simulink model "asbQuadcopter"  (R2025b)
settings: Solver=ode3  StartTime=0  StopTime=20  FixedStep=Ts  RelTol=1e-3  EnableMultiTasking=on
undefined symbols (not defined in the file): Command, ft, init, m, Rec, s, SDTV, Sim3dSensor, takeOffDuration, Ts, Vehicle
libraries: simulink x18, sim3dlib x6, aerolibconvert2 x5, aerolibsim3d x4, aerolibanimutils x2, SignalEditorBlockLib x2, environmentLibrary x2, visionconversions x2, visiongeotforms x2, visionsinks x2, sensorsLibrary x2, aerolibfltsims x2
(part 1 of 2)
settings Model: Creator=The MathWorks, Inc.  LastModifiedBy=poiuy
settings SolverCC: AlgebraicLoopSolver=TrustRegion  AutoInsertRateTranBlk=on  MaxZcPerStep=1.0
settings DataIOCC: LimitDataPoints=on  SaveFormat=Array  SaveOutput=off  DSMLogging=off  SaveTime=off  ReturnWorkspaceOutputs=off
settings OptimizationCC: BlockReduction=off  BufferReuse=off  ReuseModelBlockBuffer=off  LifeSpan=inf
settings DebuggingCC: AlgebraicLoopMsg=none  ParameterPrecisionLossMsg=none  AllowSymbolicDim=off  PregeneratedLibrarySubsystemCodeDiagnostic=none  SFUnexpectedBacktrackingDiag=warning  SFNoUnconditionalDefaultTransitionDiag=warning  SFExecutionAtInitializationDiag=none  ArithmeticOperatorsInVariantConditions=warning
settings HardwareCC: ProdBitPerPointer=32.0  ProdBitPerSizeT=32.0  ProdBitPerPtrDiffT=32.0  ProdLargestAtomicFloat=None  ProdIntDivRoundTo=Undefined  ProdEndianess=Unspecified  ProdWordSize=32.0  ProdHWDeviceType=32-bit Generic
settings ModelReferenceCC: EnableRefExpFcnMdlSchedulingChecks=on  PropagateSignalLabelsOutOfModel=off
settings SFSimCC: SimUseLocalCustomCode=off  CustomCodeUndefinedFunction=UseInterfaceOnly
settings RTWCC: RTWUseLocalCustomCode=off  GPUComputeCapability=3.5  DLArmComputeVersion=19.05
settings CodeAppCC: StateflowObjectComments=on
settings GRTTargetCC: TargetLangStandard=C89/C90 (ANSI)
settings ConfigComp: CovMetricSettings=dw  CovSaveCumulativeToWorkspaceVar=on  CovSaveSingleToWorkspaceVar=on  CovExternalEMLEnable=off  CovSFcnEnable=off

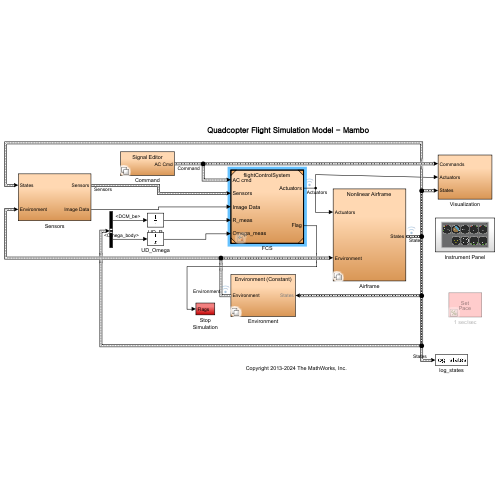
[thumbnail: Simulink's stored preview of the top-level diagram]
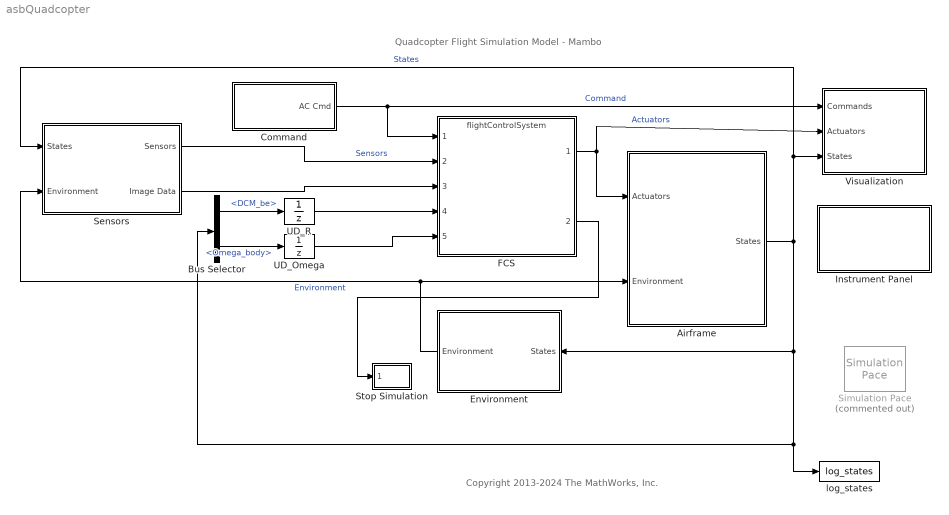
== system asbQuadcopter ==
  note: Quadcopter Flight Simulation Model - Mambo
  note: Copyright 2013-2024 The MathWorks, Inc.
  Airframe : Subsystem  Variant=on
  Bus Selector : BusSelector  OutputSignals=DCM_be,Omega_body
  Command : Subsystem  Variant=on
  Environment : Subsystem  Variant=on
  FCS : ModelReference  ModelNameDialog=flightControlSystem.slx  SimulationMode=Normal  ModelReferenceVersion=13.7
  Instrument Panel : Subsystem
  Sensors : Subsystem
  Simulation Pace : aerolibanimutils/Simulation Pace  Commented=on  SimulationPace=1  SleepMode=MATLAB Thread  OutputPaceError=off  SampleTime=Ts
      settings: AttributesFormatString=%<SimulationPace> sec/sec
  Stop Simulation : Subsystem
  UD_Omega : UnitDelay  SampleTime=0.005  HasFrameUpgradeWarning=on
  UD_R : UnitDelay  SampleTime=0.005  HasFrameUpgradeWarning=on
  Visualization : Subsystem
  log_states : ToWorkspace  VariableName=log_states  SaveFormat=Timeseries  SampleTime=-1
  wires:
  Command/1(AC Cmd) -> Visualization/1(Commands), FCS/1  "Command"
  Sensors/1(Sensors) -> FCS/2  "Sensors"
  FCS/1 -> Airframe/1(Actuators), Visualization/2(Actuators)  "Actuators"
  Environment/1(Environment) -> Sensors/2(Environment), Airframe/2(Environment)  "Environment"
  Sensors/2(Image Data) -> FCS/3
  Bus Selector/2 -> UD_Omega/1  "<Omega_body>"
  UD_Omega/1 -> FCS/5
  UD_R/1 -> FCS/4
  Bus Selector/1 -> UD_R/1  "<DCM_be>"
  FCS/2 -> Stop Simulation/1(Flags)
  Airframe/1(States) -> Environment/1(States), log_states/1, Bus Selector/1, Visualization/3(States), Sensors/1(States)  "States"

== system asbQuadcopter/Airframe ==
  note: VSS_VEHICLE = 0 will select linear airframe
      | VSS_VEHICLE = 1 will select nonlnear airframe
  Actuators : Inport
  Environment : Inport  Port=2  OutDataTypeStr=Bus: EnvironmentBus
  Linear Airframe : ModelReference  ModelNameDialog=linearAirframe.slx  SimulationMode=Normal  VariantControl=VSS_VEHICLE==DynamicsMode.Linear  ModelReferenceVersion=13.0
  Nonlinear Airframe : ModelReference  ModelNameDialog=nonlinearAirframe.slx  SimulationMode=Normal  VariantControl=VSS_VEHICLE==DynamicsMode.Nonlinear  ModelReferenceVersion=13.60
  States : Outport  OutDataTypeStr=Bus: StatesBus  VectorParamsAs1DForOutWhenUnconnected=off

== system asbQuadcopter/Command ==
  note: VSS_COMMAND = 0 will select Signal Editor
      | VSS_COMMAND = 1 will select Joystick + Signal Editor
      | VSS_COMMAND = 2 will select pre-saved data from .mat file
      | VSS_COMMAND = 3 will select pre-saved data from a spreadsheet
  Data : Subsystem  VariantControl=VSS_COMMAND==CommandMode.Presaved_data
  Joystick : Subsystem  VariantControl=VSS_COMMAND==CommandMode.Joystick
  Signal Editor : Subsystem  VariantControl=VSS_COMMAND==CommandMode.Signal_Editor
  Spreadsheet Data : Subsystem  VariantControl=VSS_COMMAND==CommandMode.Presaved_data_in_a_Spreadsheet
  AC Cmd : Outport  OutDataTypeStr=Bus: CommandBus  VectorParamsAs1DForOutWhenUnconnected=off

== system asbQuadcopter/Environment ==
  note: VSS_ENVIRONMENT = 0 will select constant environment variables
      | VSS_ENVIRONMENT = 1 will select environment variables depending on position
  States : Inport  OutDataTypeStr=Bus: StatesBus
  Environment (Constant) : environmentLibrary/Environment (Constant)  SystemSampleTime=-1  VariantControl=VSS_ENVIRONMENT==EnvironmentMode.Constant  VariantActivationTime=update diagram  EmptyChoice=off  PassThrough=off  PassThroughVariantControl=(default)  EmptyChoiceVariantControl=(default)  AllowFlexibleInterface=on  Latency=0  AutoFrameSizeCalculation=off
  Environment (Variable) : environmentLibrary/Environment (Variable)  SystemSampleTime=-1  VariantControl=VSS_ENVIRONMENT==EnvironmentMode.Variable  VariantActivationTime=update diagram  EmptyChoice=off  PassThrough=off  PassThroughVariantControl=(default)  EmptyChoiceVariantControl=(default)  AllowFlexibleInterface=on  Latency=0  AutoFrameSizeCalculation=off
  Environment : Outport  OutDataTypeStr=Bus: EnvironmentBus  VectorParamsAs1DForOutWhenUnconnected=off

== system asbQuadcopter/Instrument Panel ==
  Airspeed Indicator : AirspeedIndicatorBlock  LabelPosition=Hide  ScaleMin=0  ScaleMax=18
  Altimeter : AltimeterBlock  LabelPosition=Hide
  Artificial Horizon : ArtificialHorizonBlock  LabelPosition=Hide
  Climb Rate Indicator : ClimbIndicatorBlock  LabelPosition=Hide  ScaleMax=1000
  Heading Indicator : HeadingIndicatorBlock  LabelPosition=Hide
  Thruster {1..4} (4 alike) : RPMIndicatorBlock  LabelPosition=Hide

== system asbQuadcopter/Sensors ==
  States : Inport
  Environment : Inport  Port=2
  Camera Model : Subsystem  Variant=on
  Rate Transition3 : RateTransition  InitialCondition=zeros(4,9600)  OutPortSampleTime=VTs
  Sensor Model : Subsystem  Variant=on
  Sensors : Outport
  Image Data : Outport  Port=2
  wires:
  States/1 -> Sensor Model/1(States)
  Environment/1 -> Sensor Model/2(Environment)
  Sensor Model/1(Sensors) -> Sensors/1  "Sensors"
  Camera Model/1(image_data) -> Rate Transition3/1
  Rate Transition3/1 -> Image Data/1

== system asbQuadcopter/Stop Simulation ==
  Flags : Inport  OutDataTypeStr=uint8
  Compare To Zero : simulink/Logic and Bit Operations/Compare To Zero  relop=>  OutDataTypeStr=boolean
  Flag has been triggered : Assertion  Enabled=off
  Logical Operator : Logic  Operator=NOT  AllPortsSameDT=off  OutDataTypeStr=boolean
  wires:
  Flags/1 -> Compare To Zero/1
  Logical Operator/1 -> Flag has been triggered/1
  Compare To Zero/1 -> Logical Operator/1

== system asbQuadcopter/Visualization ==
  Commands : Inport
  Actuators : Inport  Port=2
  States : Inport  Port=3
  "Actuators " : InportShadow  Port=2
  Extract Flight Instruments : Subsystem
  "States " : InportShadow  Port=3
  Visualization : Subsystem  Variant=on
  wires:
  Actuators/1 -> Extract Flight Instruments/1(Actuators)
  States/1 -> Extract Flight Instruments/2(States)
  Commands/1 -> Visualization/2(Commands)
  "Actuators "/1 -> Visualization/3(Actuators)
  "States "/1 -> Visualization/1(States)

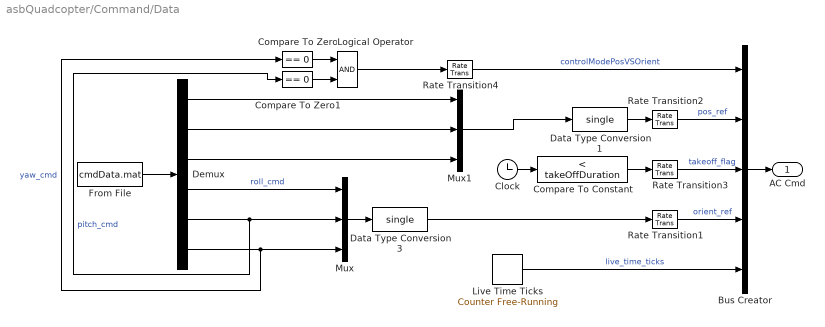
== system asbQuadcopter/Command/Data ==
  Bus Creator : BusCreator  Inputs=5  OutDataTypeStr=Bus: CommandBus  NonVirtualBus=on
  Clock : Clock
  Compare To Constant : simulink/Logic and Bit Operations/Compare To Constant  relop=<  const=takeOffDuration  OutDataTypeStr=boolean
  Compare To Zero : simulink/Logic and Bit Operations/Compare To Zero  relop===  OutDataTypeStr=boolean
  Compare To Zero1 : simulink/Logic and Bit Operations/Compare To Zero  relop===  OutDataTypeStr=boolean
  Data Type Conversion1 : DataTypeConversion  OutDataTypeStr=single  SaturateOnIntegerOverflow=off  RndMeth=Floor
  Data Type Conversion3 : DataTypeConversion  OutDataTypeStr=single  SaturateOnIntegerOverflow=off  RndMeth=Floor
  Demux : Demux  Outputs=6
  From File : FromFile  FileName=cmdData.mat  SampleTime=Ts
  Live Time Ticks : simulink/Sources/Counter Free-Running  NumBits=32  tsamp=Ts
  Logical Operator : Logic  AllPortsSameDT=off  OutDataTypeStr=boolean
  Mux : Mux  Inputs=3
  Mux1 : Mux  Inputs=3
  Rate Transition{1..4} (4 alike) : RateTransition  OutPortSampleTime=Ts
  AC Cmd : Outport  OutDataTypeStr=Bus: CommandBus  VectorParamsAs1DForOutWhenUnconnected=off
  wires:
  Demux/4 -> Mux/1  "roll_cmd"
  Demux/5 -> Mux/2, Compare To Zero1/1  "pitch_cmd"
  Demux/6 -> Compare To Zero/1, Mux/3  "yaw_cmd"
  From File/1 -> Demux/1
  Logical Operator/1 -> Rate Transition4/1
  Rate Transition1/1 -> Bus Creator/4  "orient_ref"
  Rate Transition2/1 -> Bus Creator/2  "pos_ref"
  Demux/3 -> Mux1/3
  Mux/1 -> Data Type Conversion3/1
  Data Type Conversion1/1 -> Rate Transition2/1
  Demux/1 -> Mux1/1
  Compare To Zero1/1 -> Logical Operator/2
  Compare To Zero/1 -> Logical Operator/1
  Mux1/1 -> Data Type Conversion1/1
  Clock/1 -> Compare To Constant/1
  Rate Transition4/1 -> Bus Creator/1  "controlModePosVSOrient"
  Data Type Conversion3/1 -> Rate Transition1/1
  Demux/2 -> Mux1/2
  Compare To Constant/1 -> Rate Transition3/1
  Rate Transition3/1 -> Bus Creator/3  "takeoff_flag"
  Live Time Ticks/1 -> Bus Creator/5  "live_time_ticks"
  Bus Creator/1 -> AC Cmd/1

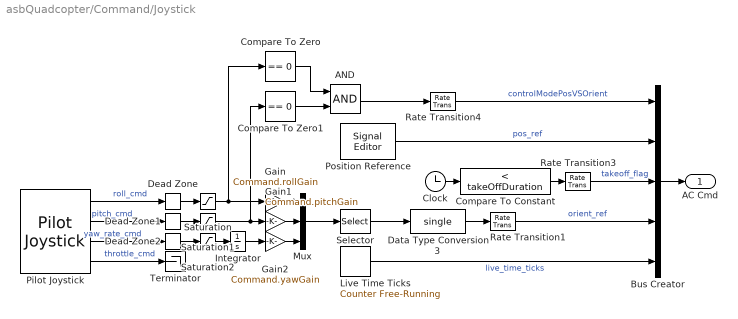
== system asbQuadcopter/Command/Joystick ==
  AND : Logic  AllPortsSameDT=off  OutDataTypeStr=boolean
  Bus Creator : BusCreator  Inputs=5  OutDataTypeStr=Bus: CommandBus  NonVirtualBus=on
  Clock : Clock
  Compare To Constant : simulink/Logic and Bit Operations/Compare To Constant  relop=<  const=takeOffDuration  OutDataTypeStr=boolean
  Compare To Zero : simulink/Logic and Bit Operations/Compare To Zero  relop===  OutDataTypeStr=boolean
  Compare To Zero1 : simulink/Logic and Bit Operations/Compare To Zero  relop===  OutDataTypeStr=boolean
  Data Type Conversion3 : DataTypeConversion  OutDataTypeStr=single  SaturateOnIntegerOverflow=off  RndMeth=Floor
  Dead Zone : DeadZone  LowerValue=Command.rollDeadZoneStart  UpperValue=Command.rollDeadZoneEnd
  Dead Zone1 : DeadZone  LowerValue=Command.pitchDeadZoneStart  UpperValue=Command.pitchDeadZoneEnd
  Dead Zone2 : DeadZone  LowerValue=Command.yawDeadZoneStart  UpperValue=Command.yawDeadZoneEnd
  Gain : Gain  Gain=Command.rollGain
  Gain1 : Gain  Gain=Command.pitchGain
  Gain2 : Gain  Gain=Command.yawGain
  Integrator : Integrator
  Live Time Ticks : simulink/Sources/Counter Free-Running  NumBits=32  tsamp=Ts
  Mux : Mux  Inputs=3
  Pilot Joystick : aerolibanimutils/Pilot Joystick  JoystickID=Joystick1  OutputConfiguration=FourAxis  SampleTime=Ts
  Position Reference : SignalEditorBlockLib/Signal Editor  FileName=positionRef.mat  ActiveScenario=Group1  ActiveSignal=XYZ  IsBus=off  OutputBusObjectStr=Bus: BusObject  SampleTime=Ts  Interpolate=off  ZeroCross=off  OutputAfterFinalValue=Setting to zero  Unit=inherit  PreserveSignalName=on  ApplySigPropsToAllScenarios=on  ApplySigPropsToAllSignals=off  SignalPropertySource=Dialog parameters
  Rate Transition1 : RateTransition  OutPortSampleTime=Ts
  Rate Transition3 : RateTransition  OutPortSampleTime=Ts
  Rate Transition4 : RateTransition  OutPortSampleTime=Ts
  Saturation : Saturate  UpperLimit=Command.rollSatUpper  LowerLimit=Command.rollSatLower
  Saturation1 : Saturate  UpperLimit=Command.pitchSatUpper  LowerLimit=Command.pitchSatLower
  Saturation2 : Saturate  UpperLimit=Command.yawSatUpper  LowerLimit=Command.yawSatLower
  Selector : Selector  InputPortWidth=3  IndexOptions=Index vector (dialog)  Indices=[3 2 1]  OutputSizes=1
  Terminator : Terminator
  AC Cmd : Outport  OutDataTypeStr=Bus: CommandBus  VectorParamsAs1DForOutWhenUnconnected=off
  wires:
  Pilot Joystick/4 -> Terminator/1  "throttle_cmd"
  Pilot Joystick/1 -> Dead Zone/1  "roll_cmd"
  Bus Creator/1 -> AC Cmd/1
  AND/1 -> Rate Transition4/1
  Rate Transition1/1 -> Bus Creator/4  "orient_ref"
  Position Reference/1 -> Bus Creator/2  "pos_ref"
  Mux/1 -> Selector/1
  Compare To Constant/1 -> Rate Transition3/1
  Clock/1 -> Compare To Constant/1
  Rate Transition4/1 -> Bus Creator/1  "controlModePosVSOrient"
  Data Type Conversion3/1 -> Rate Transition1/1
  Pilot Joystick/2 -> Dead Zone1/1  "pitch_cmd"
  Rate Transition3/1 -> Bus Creator/3  "takeoff_flag"
  Live Time Ticks/1 -> Bus Creator/5  "live_time_ticks"
  Selector/1 -> Data Type Conversion3/1
  Dead Zone/1 -> Saturation/1
  Saturation/1 -> Compare To Zero/1, Gain/1
  Gain/1 -> Mux/1
  Dead Zone1/1 -> Saturation1/1
  Saturation1/1 -> Compare To Zero1/1, Gain1/1
  Gain1/1 -> Mux/2
  Dead Zone2/1 -> Saturation2/1
  Saturation2/1 -> Integrator/1
  Gain2/1 -> Mux/3
  Pilot Joystick/3 -> Dead Zone2/1  "yaw_rate_cmd"
  Integrator/1 -> Gain2/1
  Compare To Zero/1 -> AND/1
  Compare To Zero1/1 -> AND/2

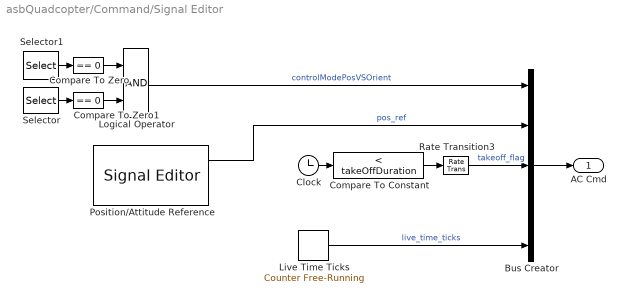
== system asbQuadcopter/Command/Signal Editor ==
  Bus Creator : BusCreator  Inputs=5  OutDataTypeStr=Bus: CommandBus  NonVirtualBus=on
  Clock : Clock
  Compare To Constant : simulink/Logic and Bit Operations/Compare To Constant  relop=<  const=takeOffDuration  OutDataTypeStr=boolean
  Compare To Zero : simulink/Logic and Bit Operations/Compare To Zero  relop===  OutDataTypeStr=boolean
  Compare To Zero1 : simulink/Logic and Bit Operations/Compare To Zero  relop===  OutDataTypeStr=boolean
  Live Time Ticks : simulink/Sources/Counter Free-Running  NumBits=32  tsamp=Ts
  Logical Operator : Logic  AllPortsSameDT=off  OutDataTypeStr=boolean
  Position/Attitude Reference : SignalEditorBlockLib/Signal Editor  FileName=positionAttitudeRef.mat  ActiveScenario=Hover  ActiveSignal=XYZ  IsBus=off  OutputBusObjectStr=Bus: BusObject  SampleTime=Ts  ZeroCross=off  OutputAfterFinalValue=Holding final value  Unit=inherit  PreserveSignalName=on  ApplySigPropsToAllScenarios=on  ApplySigPropsToAllSignals=off  SignalPropertySource=Dialog parameters
  Rate Transition3 : RateTransition  OutPortSampleTime=Ts
  Selector : Selector  InputPortWidth=3  IndexOptions=Index vector (dialog)  Indices=2  OutputSizes=1
  Selector1 : Selector  InputPortWidth=3  IndexOptions=Index vector (dialog)  Indices=3  OutputSizes=1
  AC Cmd : Outport  OutDataTypeStr=Bus: CommandBus  VectorParamsAs1DForOutWhenUnconnected=off
  wires:
  Bus Creator/1 -> AC Cmd/1
  ? -> Bus Creator/4, Selector1/1, Selector/1  "orient_ref"
  Compare To Zero/1 -> Logical Operator/1
  Compare To Zero1/1 -> Logical Operator/2
  Logical Operator/1 -> Bus Creator/1  "controlModePosVSOrient"
  Position/Attitude Reference/1 -> Bus Creator/2  "pos_ref"
  Clock/1 -> Compare To Constant/1
  Compare To Constant/1 -> Rate Transition3/1
  Rate Transition3/1 -> Bus Creator/3  "takeoff_flag"
  Live Time Ticks/1 -> Bus Creator/5  "live_time_ticks"
  Selector/1 -> Compare To Zero1/1
  Selector1/1 -> Compare To Zero/1

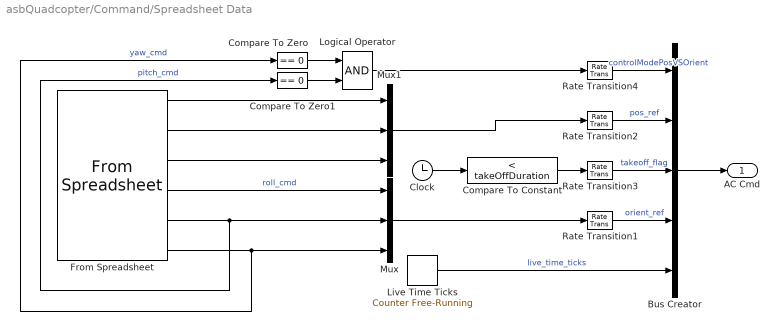
== system asbQuadcopter/Command/Spreadsheet Data ==
  Bus Creator : BusCreator  Inputs=5  OutDataTypeStr=Bus: CommandBus  NonVirtualBus=on
  Clock : Clock
  Compare To Constant : simulink/Logic and Bit Operations/Compare To Constant  relop=<  const=takeOffDuration  OutDataTypeStr=boolean
  Compare To Zero : simulink/Logic and Bit Operations/Compare To Zero  relop===  OutDataTypeStr=boolean
  Compare To Zero1 : simulink/Logic and Bit Operations/Compare To Zero  relop===  OutDataTypeStr=boolean
  From Spreadsheet : FromSpreadsheet  FileName=cmdData.xlsx  SheetName=data  OutDataTypeStr=single  SampleTime=Ts
  Live Time Ticks : simulink/Sources/Counter Free-Running  NumBits=32  tsamp=Ts
  Logical Operator : Logic  AllPortsSameDT=off  OutDataTypeStr=boolean
  Mux : Mux  Inputs=3
  Mux1 : Mux  Inputs=3
  Rate Transition{1..4} (4 alike) : RateTransition  OutPortSampleTime=Ts
  AC Cmd : Outport  OutDataTypeStr=Bus: CommandBus  VectorParamsAs1DForOutWhenUnconnected=off
  wires:
  Bus Creator/1 -> AC Cmd/1
  From Spreadsheet/4 -> Mux/1  "roll_cmd"
  From Spreadsheet/6 -> Mux/3, Compare To Zero/1  "yaw_cmd"
  Logical Operator/1 -> Rate Transition4/1
  Rate Transition1/1 -> Bus Creator/4  "orient_ref"
  Rate Transition2/1 -> Bus Creator/2  "pos_ref"
  From Spreadsheet/3 -> Mux1/3
  Mux1/1 -> Rate Transition2/1
  From Spreadsheet/1 -> Mux1/1
  Compare To Zero1/1 -> Logical Operator/2
  Compare To Zero/1 -> Logical Operator/1
  Compare To Constant/1 -> Rate Transition3/1
  Clock/1 -> Compare To Constant/1
  Rate Transition4/1 -> Bus Creator/1  "controlModePosVSOrient"
  Mux/1 -> Rate Transition1/1
  From Spreadsheet/5 -> Mux/2, Compare To Zero1/1  "pitch_cmd"
  From Spreadsheet/2 -> Mux1/2
  Rate Transition3/1 -> Bus Creator/3  "takeoff_flag"
  Live Time Ticks/1 -> Bus Creator/5  "live_time_ticks"

== system asbQuadcopter/Sensors/Camera Model ==
  note: VSS_VISUALIZATION < 3 will select Camera (Stub)
      | VSS_VISUALIZATION ==3 will select Camera (Airport)
      | VSS_VISUALIZATION ==4 will select Camera (AppleHill)
  Camera (Airport) : Subsystem  VariantControl=VSS_VISUALIZATION==3
  Camera (AppleHill) : Subsystem  VariantControl=VSS_VISUALIZATION==4
  Camera (Stub) : Subsystem  VariantControl=VSS_VISUALIZATION<3
  image_data : Outport

== system asbQuadcopter/Sensors/Sensor Model ==
  note: VSS_SENSORS = 0 will select feedthrough sensors
      | VSS_SENSORS = 1 will select dynamics sensors with noise
  States : Inport
  Environment : Inport  Port=2
  Sensors (Dynamics) : sensorsLibrary/Sensors (Dynamics)  SystemSampleTime=-1  VariantControl=VSS_SENSORS==SensorsMode.Dynamics  VariantActivationTime=update diagram  EmptyChoice=off  PassThrough=off  PassThroughVariantControl=(default)  EmptyChoiceVariantControl=(default)  AllowFlexibleInterface=on  Latency=0  AutoFrameSizeCalculation=off
  Sensors (Feedthrough) : sensorsLibrary/Sensors (Feedthrough)  SystemSampleTime=-1  VariantControl=VSS_SENSORS==SensorsMode.Feedthrough  VariantActivationTime=update diagram  EmptyChoice=off  PassThrough=off  PassThroughVariantControl=(default)  EmptyChoiceVariantControl=(default)  AllowFlexibleInterface=on  Latency=0  AutoFrameSizeCalculation=off
  Sensors : Outport  VectorParamsAs1DForOutWhenUnconnected=off

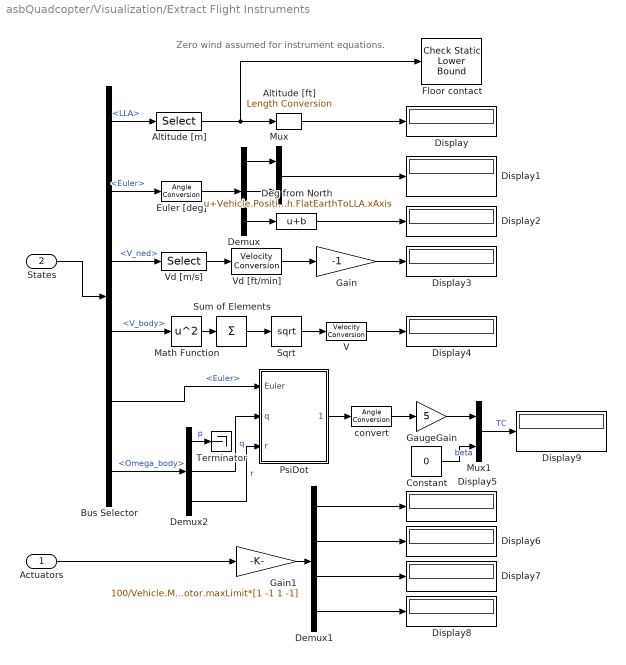
== system asbQuadcopter/Visualization/Extract Flight Instruments ==
  note: Zero wind assumed for instrument equations.
  Actuators : Inport
  States : Inport  Port=2
  Altitude [ft] : aerolibconvert2/Length Conversion  IU=m  OU=ft
  Altitude [m] : Selector  InputPortWidth=3  IndexOptions=Index vector (dialog)  Indices=[3]  OutputSizes=1
  Bus Selector : BusSelector  OutputSignals=LLA,Euler,V_ned,V_body,Euler,Omega_body
  Constant : Constant  Value=0
  Deg from North : Bias  Bias=Vehicle.PositionOnEarth.FlatEarthToLLA.xAxis  SaturateOnIntegerOverflow=off
  Demux : Demux  Outputs=3
  Demux1 : Demux
  Demux2 : Demux  Outputs=3
  Display{,1..9} (10 alike) : Display
  Euler [deg] : aerolibconvert2/Angle Conversion  IU=rad  OU=deg
  Floor contact : simulink/Model Verification/Check Static  Lower Bound  Description=init.posLLA(3) <= u  min=init.posLLA(3)  min_included=on  enabled=on  stopWhenAssertionFail=on  export=off  icon=graphic
  Gain : Gain  Gain=-1
  Gain1 : Gain  Gain=100/Vehicle.Motor.maxLimit*[1 -1 1 -1]
  GaugeGain : Gain  Gain=5
  Math Function : Math  Operator=square  SignedPower=on
  Mux : Mux  Inputs=2
  Mux1 : Mux  Inputs=2
  PsiDot : Subsystem
  Sqrt : Sqrt
  Sum of Elements : Sum  Inputs=+
  Terminator : Terminator
  V : aerolibconvert2/Velocity Conversion  IU=m/s  OU=kts
  Vd [ft/min] : aerolibconvert2/Velocity Conversion  IU=m/s  OU=ft/min
  Vd [m/s] : Selector  InputPortWidth=3  IndexOptions=Index vector (dialog)  Indices=[3]  OutputSizes=1
  convert : aerolibconvert2/Angle Conversion  IU=rad  OU=deg
  wires:
  Bus Selector/1 -> Altitude [m]/1  "<LLA>"
  Altitude [m]/1 -> Floor contact/1, Altitude [ft]/1
  States/1 -> Bus Selector/1
  Altitude [ft]/1 -> Display/1
  Bus Selector/2 -> Euler [deg]/1  "<Euler>"
  Euler [deg]/1 -> Demux/1
  Demux/1 -> Mux/1
  Demux/2 -> Mux/2
  Mux/1 -> Display1/1
  Deg from North/1 -> Display2/1
  Bus Selector/3 -> Vd [m/s]/1  "<V_ned>"
  Vd [m/s]/1 -> Vd [ft/min]/1
  Vd [ft/min]/1 -> Gain/1
  Gain/1 -> Display3/1
  Math Function/1 -> Sum of Elements/1
  Sum of Elements/1 -> Sqrt/1
  Bus Selector/4 -> Math Function/1  "<V_body>"
  Sqrt/1 -> V/1
  V/1 -> Display4/1
  Gain1/1 -> Demux1/1
  Demux1/1 -> Display5/1
  Demux1/2 -> Display6/1
  Demux1/3 -> Display7/1
  Demux1/4 -> Display8/1
  Actuators/1 -> Gain1/1
  Demux/3 -> Deg from North/1
  Mux1/1 -> Display9/1  "TC"
  Constant/1 -> Mux1/2  "beta"
  Bus Selector/6 -> Demux2/1  "<Omega_body>"
  Demux2/1 -> Terminator/1  "p"
  Demux2/2 -> PsiDot/2(q)  "q"
  Demux2/3 -> PsiDot/3(r)  "r"
  PsiDot/1(psi_dot) -> convert/1
  convert/1 -> GaugeGain/1
  GaugeGain/1 -> Mux1/1
  Bus Selector/5 -> PsiDot/1(Euler)  "<Euler>"

== system asbQuadcopter/Visualization/Visualization ==
  note: VSS_VISUALIZATION = 0 will select scopes as means to visualize variables/states
      | VSS_VISUALIZATION = 1 will send select states in a variable to the workspace
      | VSS_VISUALIZATION = 2 will use FlightGear as visualization
      | VSS_VISUALIZATION = 3 will use the Airport Scene in the Unreal Engine environment
      | VSS_VISUALIZATION = 4 will use the Apple Hill Scene in the Unreal Engine environment
  States : Inport  OutDataTypeStr=Bus: StatesBus
  Commands : Inport  Port=2  OutDataTypeStr=Bus: CommandBus
  Actuators : Inport  Port=3
  AirportScene : Subsystem  VariantControl=VSS_VISUALIZATION==VisualizationMode.AirportScene
  AppleHillScene : Subsystem  VariantControl=VSS_VISUALIZATION==VisualizationMode.AppleHillScene
  FlightGear : Subsystem  VariantControl=VSS_VISUALIZATION==VisualizationMode.FlightGear
      mask init:
      | visualizationFlightGearVars;
  Scopes : Subsystem  VariantControl=VSS_VISUALIZATION==VisualizationMode.Scopes
  Workspace : Subsystem  VariantControl=VSS_VISUALIZATION==VisualizationMode.Send_values_to_workspace

== system asbQuadcopter/Sensors/Camera Model/Camera (Airport) ==
  RGB to Y1UY2V1 : Subsystem
  Rotate : visiongeotforms/Rotate  outSizeR=Expanded to fit rotated input image  src_angle=Specify via dialog  unit_angle=Degrees  angle=pi/2  maxAngle=pi  dispImage=Top-left corner  method=Table lookup  fillVal=0  interpMethod=Bilinear  roundingMode=Nearest  overflowMode=on  prodOutputMode=Binary point scaling  prodOutputWordLength=32  prodOutputFracLength=10
  Simulation 3D Camera Get : sim3dlib/Simulation 3D Camera Get  Priority=1  sensorTag=Sim3dSensor�  sensorId=1  sensorName=Sim3dSensor�  vehTagList={'Scene Origin';'Sim3dActorAirport';'Sim3dActorAppleHill';'SimulinkVehicleAirport';'SimulinkVehicleAppleHill'}  vehTag=SimulinkVehicleAirport  CoordinateSystem=ISO8855  mountLoc=Down  offsetFlag=off  tmountOffset=[0, 0, 0]  rmountOffset=[0, 0, 0]  HorizontalResolution=120  VerticalResolution=160  HorizontalFOV=90  SampleTime=-1  mountPoint=[0 0 0.03]  mountOrientation=[0 90 0]  aMode=0  ID=1
      settings: LibrarySourceBlock=aerolibsim3d/Simulation 3D Camera Get
  To Video Display : visionsinks/To Video Display  windowSizeMode=Normal  openAtMdlStart=on  fullScreen=off  videoWindowX=536805376  videoWindowY=536805376  saveWindowSize=off  videoWindowWidth=236  videoWindowHeight=160  inputColorFormat=RGB  inputType=Obsolete  imagePorts=One multidimensional signal  OutputDevice=On-screen video monitor  dataOrg=Column-major  isWindowOpen=off
  image_data : Outport
  wires:
  Simulation 3D Camera Get/1 -> Rotate/1, To Video Display/1
  RGB to Y1UY2V1/1(Y1UY2VImage) -> image_data/1
  Rotate/1 -> RGB to Y1UY2V1/1(RGBImage)

== system asbQuadcopter/Sensors/Camera Model/Camera (AppleHill) ==
  RGB to Y1UY2V1 : Subsystem
  Rotate : visiongeotforms/Rotate  outSizeR=Expanded to fit rotated input image  src_angle=Specify via dialog  unit_angle=Degrees  angle=pi/2  maxAngle=pi  dispImage=Top-left corner  method=Table lookup  fillVal=0  interpMethod=Bilinear  roundingMode=Nearest  overflowMode=on  prodOutputMode=Binary point scaling  prodOutputWordLength=32  prodOutputFracLength=10
  Simulation 3D Camera Get : sim3dlib/Simulation 3D Camera Get  Priority=1  sensorTag=Sim3dSensor�  sensorId=2  sensorName=Sim3dSensor�  vehTagList={'Scene Origin';'Sim3dActorAirport';'Sim3dActorAppleHill';'SimulinkVehicleAirport';'SimulinkVehicleAppleHill'}  vehTag=SimulinkVehicleAppleHill  CoordinateSystem=ISO8855  mountLoc=Down  offsetFlag=off  tmountOffset=[0, 0, 0]  rmountOffset=[0, 0, 0]  HorizontalResolution=120  VerticalResolution=160  HorizontalFOV=90  SampleTime=-1  mountPoint=[0 0 0]  mountOrientation=[0 0 0]  aMode=0  ID=2
      settings: LibrarySourceBlock=aerolibsim3d/Simulation 3D Camera Get
  To Video Display : visionsinks/To Video Display  windowSizeMode=Normal  openAtMdlStart=on  fullScreen=off  videoWindowX=536805376  videoWindowY=536805376  saveWindowSize=off  videoWindowWidth=2147483647  videoWindowHeight=2147483647  inputColorFormat=RGB  inputType=Obsolete  imagePorts=One multidimensional signal  OutputDevice=On-screen video monitor  dataOrg=Column-major  isWindowOpen=off
  image_data : Outport
  wires:
  RGB to Y1UY2V1/1(Y1UY2VImage) -> image_data/1
  Rotate/1 -> RGB to Y1UY2V1/1(RGBImage)
  Simulation 3D Camera Get/1 -> Rotate/1, To Video Display/1

== system asbQuadcopter/Sensors/Camera Model/Camera (Stub) ==
  Constant : Constant  Value=zeros(4,9600)  OutDataTypeStr=uint8
  image_data : Outport
  wires:
  Constant/1 -> image_data/1

== system asbQuadcopter/Visualization/Extract Flight Instruments/PsiDot ==
  Euler : Inport
  q : Inport  Port=2
  r : Inport  Port=3
  Add : Sum
  Cos : Trigonometry  Operator=cos
  Cos1 : Trigonometry  Operator=cos
  Demux : Demux  Outputs=3
  Product : Product  Inputs=**/
  Product1 : Product  Inputs=**/
  Sin : Trigonometry
  Terminator : Terminator
  psi_dot : Outport
  wires:
  Demux/2 -> Cos/1  "theta"
  Add/1 -> psi_dot/1
  Cos/1 -> Product/3, Product1/3
  q/1 -> Product1/2
  r/1 -> Product/2
  Product1/1 -> Add/1
  Product/1 -> Add/2
  Demux/1 -> Cos1/1, Sin/1  "phi"
  Sin/1 -> Product1/1
  Cos1/1 -> Product/1
  Demux/3 -> Terminator/1
  Euler/1 -> Demux/1

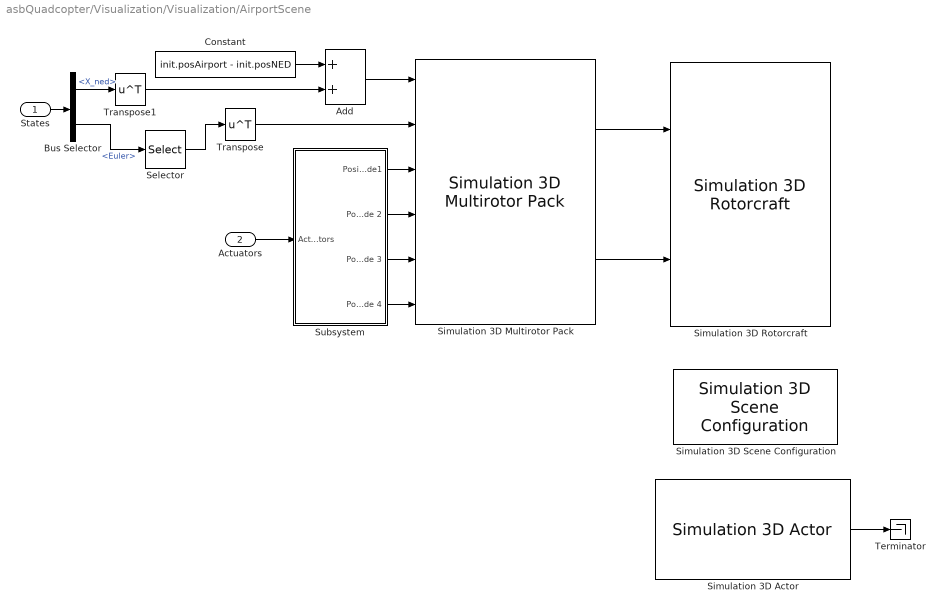
== system asbQuadcopter/Visualization/Visualization/AirportScene ==
  States : Inport
  Actuators : Inport  Port=2
  Add : Sum
  Bus Selector : BusSelector  OutputSignals=X_ned,Euler
  Constant : Constant  Value=init.posAirport - init.posNED
  Selector : Selector  InputPortWidth=3  IndexOptions=Index vector (dialog)  Indices=[3 2 1]  OutputSizes=1
  Simulation 3D Actor : sim3dlib/Simulation 3D Actor  ActorName=Sim3dActorAirport  ParentName=Scene Origin  Operation=Create at setup  InitScriptText=|  SampleTime=-1  Translation=single([0 0 0])  Rotation=single([0 0 0])  Scale=single([1 1 1])  aMode=5  ActorTag=Sim3dActorAirport  ActorType=Sim3dActor  ID=C
      | % Units are in meters
      | block = sim3d.Actor('ActorName', 'Target');
      | block.createShape('box', [.5 .5 .3]);
      | block.Color = [1 0 0];  % red
      | initPos = evalin('base','init.posAirportActor');
      | block.Translation = initPos;  % resting on the ground
      | World.add(block, Actor);
      settings: LibrarySourceBlock=sl3dlib/Simulation 3D/Simulation 3D Actor
  Simulation 3D Multirotor Pack : aerolibsim3d/Simulation 3D Multirotor Pack  Rotor1_T=off  Rotor1_R=on  Rotor2_T=off  Rotor2_R=on  Rotor3_T=off  Rotor3_R=on  Rotor4_T=off  Rotor4_R=on  Rotor5_T=off  Rotor5_R=off  Rotor6_T=off  Rotor6_R=off  Rotor7_T=off  Rotor7_R=off  Rotor8_T=off  Rotor8_R=off  Sensor1_T=off  Sensor1_R=off  Sensor2_T=off  Sensor2_R=off  EnableUETransform=on  GeoRadioButton=NED
      settings: AttributesFormatString=NED
  Simulation 3D Rotorcraft : aerolibsim3d/Simulation 3D Rotorcraft  Priority=-1  Mesh=Multirotor  MeshPath=/MathWorksAerospaceContent/Vehicles/Rotorcraft/Helicopter/Mesh/SK_Helicopter.SK_Helicopter  MeshPathLight=/MathWorksAerospaceContent/Vehicles/Rotorcraft/LightHelicopter/Mesh/SK_LightHelicopter.SK_LightHelicopter  MeshPathMulti=/MathWorksAerospaceContent/Vehicles/Rotorcraft/Multirotor/Mesh/SK_Quadcopter.SK_Quadcopter  AircraftColor=Red  ActorName=SimulinkVehicleAirport  Translation=[init.posAirport; zeros(10, 3)]  Rotation=zeros(11, 3)  ScaleInputPort=Dialog  Scale=[1 1 1]  InitialScale=[1 1 1]  IsGHSensorEnabled=off  AreGHRaysVisible=off  IsOutputReshapeEnabled=off  GHRayLength=1524  GHBodyOffset=1.169  GHFrontTireRadius=0.196  GHLeftTireRadius=0.203  GHRightTireRadius=0.203  GHContactLocation1=[1.47 -1.04 1.169]  GHContactLocation2=[-1.24 -1.04 1.169]  GHContactLocation3=[-1.24 1.04 1.169]  GHContactLocation4=[1.47 1.04 1.169]  WoWSensorTolerance=0.05  LightsConfig=Automatic lights  LandingLightIntensity=300000  LandingLightConeAngle=15  LandingLightColor=[1 1 1]  HelicopterLeftLandingLightLocation=[0 0 0]  HelicopterLeftLandingLightOrientation=[0 0 0]  NoseLightIntensity=150000  NoseLightConeAngle=36  HelicopterNoseLightLocation=[0 0 0]  HelicopterNoseLightOrientation=[0 0 0]  NavLightIntensity=500  PositionLightIntensity=500  StrobeLightIntensity=5000  StrobeLightColor=[1 1 1]  StrobePeriod=1.5  StrobePulseWidth=6  BeaconLightIntensity=4000  BeaconLightColor=[1 0 0]  BeaconPeriod=1.5  BeaconPulseWidth=10  SampleTime=-1  ActorType=SimulinkVehicle  ID=C  aMode=0  ActorTag=SimulinkVehicleAirport
  Simulation 3D Scene Configuration : sim3dlib/Simulation 3D Scene Configuration  Priority=0  ProjectFormat=Default Scenes  SceneDesc=Airport  ProjectName=C:\Program Files\MATLAB\R2025b\toolbox\shared\sim3d_projects\automotive_project_windows\UE\WindowsNoEditor\VehicleSimulation.exe  ScenePath=/Game/Maps/HwStrght  EnableOpenDRIVE=off  vehTagList={'Custom';'Scene Origin';'Sim3dActorAirport';'SimulinkVehicleAirport'}  vehTag=Custom  AttachedCameraRelativeTranslation=[0 0 0]  FreeCameraDefaultInitialTranslation=[-6, 0, 2]  AttachedCameraRelativeRotation=[0 0 0]  FreeCameraDefaultInitialRotation=[0, -15, 0]  ViewpointName=Custom  FreeCameraInitialTranslation=[3900 -4 1]  ViewpointTranslation=[0 0 0]  FreeCameraInitialRotation=[0 0 90]  ViewpointRotation=[0 0 0]  OpVisEn=off  Ts=.02  EnableWindow=on  EnableRemoteAccess=off  EnableWeather=off  SunAzimuth=90  SunAltitude=40.0  EnableGeospatialSun=off  Latitude=0  Longitude=0  Date=2023-01-01  Time=10:30:00  GeoTimeZone=-5.0  SunDaylightSaving=off  wind=1  clouds=10  EnableVolumetricClouds=off  CloudCoverage=0  CloudAltitude=6  fog=0  rain=0  RaindropsEffect=off  SnowDensity=0  EnableGeospatial=off  TilesetSource=Earth terrain  UseTrueOrigin=off  OriginHeight=200  OriginLatitude=40.744652  OriginLongitude=-73.988864  MapStyle=Aerial  AdditionalAssetIDs=[]  UseAdvancedSunSky=off  SolarTime=11  TimeZone=-5  Day=21  Month=9  Year=2022  UseDaylightSavingTime=on  DSTStartDay=10  DSTStartMonth=3  DSTEndDay=3  DSTEndMonth=11  DSTSwitchHour=2  sensorTag=MainCamera1  sensorId=1  sensorName=MainCamera1  mountLoc=Origin  offsetFlag=off  tmountOffset=[0, 0, 0]  rmountOffset=[0, 0, 0]  HorizontalResolution=1280  VerticalResolution=720  HorizontalFOV=60  mountPoint=[0 0 0]  mountOrientation=[0 0 0]  aMode=0  ID=1  GeoTrigger=Inactive  ViewNameList={'Custom'}  ViewTranslationList={'[3900 -4 1]'}  ViewRotationList={'[0 0 90]'}
      settings: AttributesFormatString=NED  LibrarySourceBlock=aerolibsim3d/Simulation 3D Scene Configuration
  Subsystem : Subsystem
  Terminator : Terminator
  Transpose : Math  Operator=transpose
  Transpose1 : Math  Operator=transpose
  wires:
  Simulation 3D Actor/1 -> Terminator/1
  Simulation 3D Multirotor Pack/2 -> Simulation 3D Rotorcraft/2
  Subsystem/1(Position Blade1) -> Simulation 3D Multirotor Pack/3
  States/1 -> Bus Selector/1
  Bus Selector/1 -> Transpose1/1  "<X_ned>"
  Simulation 3D Multirotor Pack/1 -> Simulation 3D Rotorcraft/1
  Subsystem/3(Position Blade 3) -> Simulation 3D Multirotor Pack/5
  Transpose/1 -> Simulation 3D Multirotor Pack/2
  Actuators/1 -> Subsystem/1(Actuators)
  Subsystem/4(Position Blade 4) -> Simulation 3D Multirotor Pack/6
  Transpose1/1 -> Add/2
  Subsystem/2(Position Blade 2) -> Simulation 3D Multirotor Pack/4
  Constant/1 -> Add/1
  Add/1 -> Simulation 3D Multirotor Pack/1
  Bus Selector/2 -> Selector/1  "<Euler>"
  Selector/1 -> Transpose/1

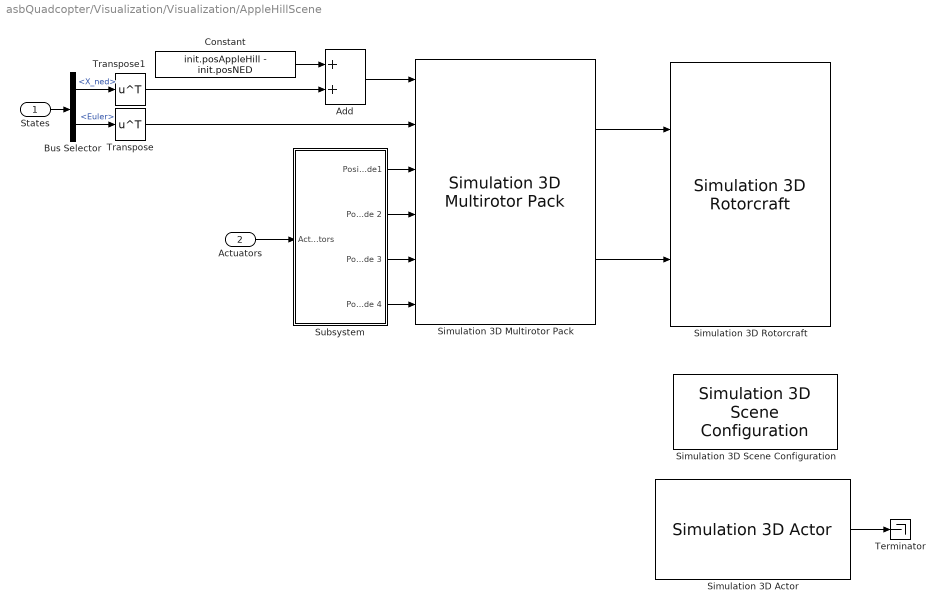
== system asbQuadcopter/Visualization/Visualization/AppleHillScene ==
  States : Inport
  Actuators : Inport  Port=2
  Add : Sum
  Bus Selector : BusSelector  OutputSignals=X_ned,Euler
  Constant : Constant  Value=init.posAppleHill - init.posNED
  Simulation 3D Actor : sim3dlib/Simulation 3D Actor  ActorName=Sim3dActorAppleHill  ParentName=Scene Origin  Operation=Create at setup  InitScriptText=|  SampleTime=-1  Translation=single([0 0 0])  Rotation=single([0 0 0])  Scale=single([1 1 1])  aMode=5  ActorTag=Sim3dActorAppleHill  ActorType=Sim3dActor  ID=C
      | % Units are in meters
      | block = sim3d.Actor('ActorName', 'Target');
      | block.createShape('box', [.5 .5 .3]);
      | block.Color = [1 0 0];  % red
      | initPos = evalin('base','init.posAppleHillActor');
      | block.Translation = initPos;  % resting on the ground
      | World.add(block, Actor);
      settings: LibrarySourceBlock=sl3dlib/Simulation 3D/Simulation 3D Actor
  Simulation 3D Multirotor Pack : aerolibsim3d/Simulation 3D Multirotor Pack  Rotor1_T=off  Rotor1_R=on  Rotor2_T=off  Rotor2_R=on  Rotor3_T=off  Rotor3_R=on  Rotor4_T=off  Rotor4_R=on  Rotor5_T=off  Rotor5_R=off  Rotor6_T=off  Rotor6_R=off  Rotor7_T=off  Rotor7_R=off  Rotor8_T=off  Rotor8_R=off  Sensor1_T=off  Sensor1_R=off  Sensor2_T=off  Sensor2_R=off  EnableUETransform=on  GeoRadioButton=NED
      settings: AttributesFormatString=NED
  Simulation 3D Rotorcraft : aerolibsim3d/Simulation 3D Rotorcraft  Priority=-1  Mesh=Multirotor  MeshPath=/MathWorksAerospaceContent/Vehicles/Rotorcraft/Helicopter/Mesh/SK_Helicopter.SK_Helicopter  MeshPathLight=/MathWorksAerospaceContent/Vehicles/Rotorcraft/LightHelicopter/Mesh/SK_LightHelicopter.SK_LightHelicopter  MeshPathMulti=/MathWorksAerospaceContent/Vehicles/Rotorcraft/Multirotor/Mesh/SK_Quadcopter.SK_Quadcopter  AircraftColor=Red  ActorName=SimulinkVehicleAppleHill  Translation=[init.posAppleHill; zeros(10, 3)]  Rotation=zeros(11, 3)  ScaleInputPort=Dialog  Scale=[1 1 1]  InitialScale=[1 1 1]  IsGHSensorEnabled=off  AreGHRaysVisible=off  IsOutputReshapeEnabled=off  GHRayLength=1524  GHBodyOffset=1.169  GHFrontTireRadius=0.196  GHLeftTireRadius=0.203  GHRightTireRadius=0.203  GHContactLocation1=[1.47 -1.04 1.169]  GHContactLocation2=[-1.24 -1.04 1.169]  GHContactLocation3=[-1.24 1.04 1.169]  GHContactLocation4=[1.47 1.04 1.169]  WoWSensorTolerance=0.05  LightsConfig=Automatic lights  LandingLightIntensity=300000  LandingLightConeAngle=15  LandingLightColor=[1 1 1]  HelicopterLeftLandingLightLocation=[0 0 0]  HelicopterLeftLandingLightOrientation=[0 0 0]  NoseLightIntensity=150000  NoseLightConeAngle=36  HelicopterNoseLightLocation=[0 0 0]  HelicopterNoseLightOrientation=[0 0 0]  NavLightIntensity=500  PositionLightIntensity=500  StrobeLightIntensity=5000  StrobeLightColor=[1 1 1]  StrobePeriod=1.5  StrobePulseWidth=6  BeaconLightIntensity=4000  BeaconLightColor=[1 0 0]  BeaconPeriod=1.5  BeaconPulseWidth=10  SampleTime=-1  ActorType=SimulinkVehicle  ID=C  aMode=0  ActorTag=SimulinkVehicleAppleHill
  Simulation 3D Scene Configuration : sim3dlib/Simulation 3D Scene Configuration  Priority=0  ProjectFormat=Unreal Editor  SceneDesc=Airport  ProjectName=Z:\41\ssivadas.Bdoc24a.j2482140\matlab\toolbox\shared\sim3d_projects\automotive_project_windows\UE\WindowsNoEditor\VehicleSimulation.exe  ScenePath=/Game/Maps/HwStrght  UEProjPath=C:\Local\AutoVrtlEnv\AutoVrtlEnv.uproject  EnableOpenDRIVE=off  vehTagList={'Custom';'Scene Origin';'Sim3dActorAirport';'Sim3dActorAppleHill';'SimulinkVehicleAirport';'SimulinkVehicleAppleHill'}  vehTag=SimulinkVehicleAppleHill  AttachedCameraRelativeTranslation=[0 0 0]  FreeCameraDefaultInitialTranslation=[-6, 0, 2]  AttachedCameraRelativeRotation=[0 0 0]  FreeCameraDefaultInitialRotation=[0, -15, 0]  ViewpointName=Custom  FreeCameraInitialTranslation=[-6, 0, 2]  ViewpointTranslation=[0 0 0]  FreeCameraInitialRotation=[0, -15, 0]  ViewpointRotation=[0 0 0]  OpVisEn=off  Ts=.02  EnableWindow=on  EnableRemoteAccess=off  EnableWeather=off  SunAzimuth=90  SunAltitude=40.0  EnableGeospatialSun=off  Latitude=0  Longitude=0  Date=2023-01-01  Time=10:30:00  GeoTimeZone=-5.0  SunDaylightSaving=off  wind=1  clouds=10  EnableVolumetricClouds=off  CloudCoverage=0  CloudAltitude=6  fog=0  rain=0  RaindropsEffect=off  SnowDensity=0  EnableGeospatial=off  TilesetSource=Earth terrain  UseTrueOrigin=off  OriginHeight=200  OriginLatitude=40.744652  OriginLongitude=-73.988864  MapStyle=Aerial  AdditionalAssetIDs=[]  UseAdvancedSunSky=off  SolarTime=11  TimeZone=-5  Day=21  Month=9  Year=2022  UseDaylightSavingTime=on  DSTStartDay=10  DSTStartMonth=3  DSTEndDay=3  DSTEndMonth=11  DSTSwitchHour=2  sensorTag=MainCamera2  sensorId=2  sensorName=MainCamera2  mountLoc=Origin  offsetFlag=off  tmountOffset=[0, 0, 0]  rmountOffset=[0, 0, 0]  HorizontalResolution=1280  VerticalResolution=720  HorizontalFOV=60  mountPoint=[0 0 0]  mountOrientation=[0 0 0]  aMode=0  ID=2  GeoTrigger=Inactive  ViewNameList={'Custom'}  ViewTranslationList={'[-6 0 2]'}  ViewRotationList={'[0 -15 0]'}
      settings: LibrarySourceBlock=aerolibsim3d/Simulation 3D Scene Configuration
  Subsystem : Subsystem
  Terminator : Terminator
  Transpose : Math  Operator=transpose
  Transpose1 : Math  Operator=transpose
  wires:
  Add/1 -> Simulation 3D Multirotor Pack/1
  Bus Selector/1 -> Transpose1/1  "<X_ned>"
  Simulation 3D Multirotor Pack/1 -> Simulation 3D Rotorcraft/1
  Simulation 3D Multirotor Pack/2 -> Simulation 3D Rotorcraft/2
  Constant/1 -> Add/1
  Subsystem/1(Position Blade1) -> Simulation 3D Multirotor Pack/3
  Transpose1/1 -> Add/2
  Transpose/1 -> Simulation 3D Multirotor Pack/2
  Subsystem/3(Position Blade 3) -> Simulation 3D Multirotor Pack/5
  States/1 -> Bus Selector/1
  Simulation 3D Actor/1 -> Terminator/1
  Subsystem/4(Position Blade 4) -> Simulation 3D Multirotor Pack/6
  Actuators/1 -> Subsystem/1(Actuators)
  Bus Selector/2 -> Transpose/1  "<Euler>"
  Subsystem/2(Position Blade 2) -> Simulation 3D Multirotor Pack/4

== system asbQuadcopter/Visualization/Visualization/FlightGear ==
  States : Inport
  Bus Selector : BusSelector  OutputSignals=LLA,Euler
  FlightGear Preconfigured 6DoF Animation : aerolibfltsims/FlightGear Preconfigured 6DoF Animation  xFlightGearVersion=v2019.1  DestinationIpAddress=127.0.0.1  DestinationPort=Visualization.FlightGear.SixDOF.destinationPort  SampleTime=Ts  packetVersion=24
  Generate Run Script : aerolibfltsims/Generate Run Script  Architecture=Default  dataFlow=Send  GeometryModelName=Model  AirportId=KSFO  RunwayId=10L  InitialAltitude=Visualization.FlightGear.generateRunScript.initialAltitude  InitialHeading=Visualization.FlightGear.generateRunScript.initialHeading  OffsetDistance=Visualization.FlightGear.generateRunScript.offsetDistance  OffsetAzimuth=Visualization.FlightGear.generateRunScript.offsetAzimuth  InstallScenery=off  DisableShaders=off  OriginAddress=127.0.0.1  DestinationPort=Visualization.FlightGear.generateRunScript.destinationPort  OriginPort=5505  LocalAddress=127.0.0.1  OutputFileName=runfg.bat  FlightGearBaseDirectory=C:\Program Files\FlightGear
  Math Function : Math  Operator=transpose  SignedPower=on
  Mux : Mux  Inputs=2
  wires:
  States/1 -> Bus Selector/1
  Bus Selector/2 -> Mux/2  "<Euler>"
  Mux/1 -> FlightGear Preconfigured 6DoF Animation/1
  Bus Selector/1 -> Math Function/1  "<LLA>"
  Math Function/1 -> Mux/1

== system asbQuadcopter/Visualization/Visualization/Scopes ==
  Commands : Inport
  States : Inport  Port=2
  Bus Creator : BusCreator  Inputs=2
  Bus Selector : BusSelector  OutputSignals=States.V_body,States.Euler,States.X_ned
  Euler : Scope
      settings: ActiveDisplayYMinimum=-0.0140044  ActiveDisplayYMaximum=0.125876  DataLoggingVariableName=ScopeData2
  V_body : Scope
      settings: ActiveDisplayYMinimum=-2.96824  ActiveDisplayYMaximum=14.7064
  X_ned : Scope
      settings: ActiveDisplayYMinimum=-0.0140044  ActiveDisplayYMaximum=0.125876
  wires:
  Commands/1 -> Bus Creator/1  "Commands"
  States/1 -> Bus Creator/2  "States"
  Bus Creator/1 -> Bus Selector/1
  Bus Selector/1 -> V_body/1  "<V_body>"
  Bus Selector/2 -> Euler/1  "<Euler>"
  Bus Selector/3 -> X_ned/1  "<X_ned>"

== system asbQuadcopter/Visualization/Visualization/Workspace ==
  Commands : Inport
  States : Inport  Port=2
  Bus Selector : BusSelector  OutputSignals=V_body,Omega_body,Euler
  Bus Selector1 : BusSelector  OutputSignals=controlModePosVSOrient,pos_ref,takeoff_flag,orient_ref
  CommandsOut : ToWorkspace  VariableName=CommandsOut  SaveFormat=Structure With Time  SampleTime=-1
  Data Type Conversion{,1..3} (4 alike) : DataTypeConversion  OutDataTypeStr=double  SaturateOnIntegerOverflow=off  RndMeth=Floor
  Mux : Mux  Inputs=3
  Mux1 : Mux
  StatesOut : ToWorkspace  VariableName=statesOut  SaveFormat=Structure With Time  SampleTime=-1
  wires:
  States/1 -> Bus Selector/1
  Bus Selector/2 -> Mux/2  "<Omega_body>"
  Bus Selector/3 -> Mux/3  "<Euler>"
  Bus Selector/1 -> Mux/1  "<V_body>"
  Mux/1 -> StatesOut/1
  Commands/1 -> Bus Selector1/1
  Bus Selector1/2 -> Data Type Conversion1/1  "<pos_ref>"
  Bus Selector1/1 -> Data Type Conversion/1  "<controlModePosVSOrient>"
  Mux1/1 -> CommandsOut/1
  Bus Selector1/4 -> Data Type Conversion3/1  "<orient_ref>"
  Bus Selector1/3 -> Data Type Conversion2/1  "<takeoff_flag>"
  Data Type Conversion/1 -> Mux1/1
  Data Type Conversion1/1 -> Mux1/2
  Data Type Conversion2/1 -> Mux1/3
  Data Type Conversion3/1 -> Mux1/4

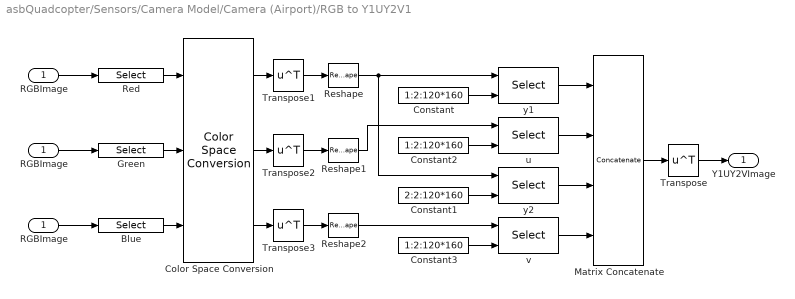
== system asbQuadcopter/Sensors/Camera Model/Camera (Airport)/RGB to Y1UY2V1 ==
  RGBImage : Inport  OutDataTypeStr=uint8  PortDimensions=[120 160 3]
  " RGBImage " : InportShadow  OutDataTypeStr=uint8  PortDimensions=[120 160 3]
  Blue : Selector  NumberOfDimensions=3  InputPortWidth=3  IndexOptions=Select all,Select all,Index vector (dialog)  Indices=1,1,3  OutputSizes=1,1,1
  Color Space Conversion : visionconversions/Color Space  Conversion  conversion=Obsolete  conversionActive=R'G'B' to Y'CbCr  wp_str=D65  rec=Rec. 601 (SDTV)  sys=1125/60/2:1  imagePorts=Separate color signals
  Constant : Constant  Value=1:2:120*160
  Constant1 : Constant  Value=2:2:120*160
  Constant2 : Constant  Value=1:2:120*160
  Constant3 : Constant  Value=1:2:120*160
  Green : Selector  NumberOfDimensions=3  InputPortWidth=3  IndexOptions=Select all,Select all,Index vector (dialog)  Indices=1,1,2  OutputSizes=1,1,1
  Matrix Concatenate : Concatenate  NumInputs=4  Mode=Multidimensional array  ConcatenateDimension=2
  "RGBImage " : InportShadow  OutDataTypeStr=uint8  PortDimensions=[120 160 3]
  Red : Selector  NumberOfDimensions=3  InputPortWidth=3  IndexOptions=Select all,Select all,Index vector (dialog)  Indices=1,1,1  OutputSizes=1,1,1
  Reshape : Reshape
  Reshape1 : Reshape
  Reshape2 : Reshape
  Transpose{,1..3} (4 alike) : Math  Operator=transpose  SignedPower=on
  u : Selector  InputPortWidth=120*160  IndexOptions=Index vector (port)  Indices=[1 3]  OutputSizes=1
  v : Selector  InputPortWidth=120*160  IndexOptions=Index vector (port)  Indices=[1 3]  OutputSizes=1
  y1 : Selector  InputPortWidth=120*160  IndexOptions=Index vector (port)  Indices=[1 3]  OutputSizes=1
  y2 : Selector  InputPortWidth=120*160  IndexOptions=Index vector (port)  Indices=[1 3]  OutputSizes=1
  Y1UY2VImage : Outport  OutDataTypeStr=uint8  PortDimensions=[4 9600]  VectorParamsAs1DForOutWhenUnconnected=off
  wires:
  Matrix Concatenate/1 -> Transpose/1
  v/1 -> Matrix Concatenate/4
  y1/1 -> Matrix Concatenate/1
  RGBImage/1 -> Green/1
  Color Space Conversion/2 -> Transpose2/1
  Color Space Conversion/1 -> Transpose1/1
  Color Space Conversion/3 -> Transpose3/1
  Red/1 -> Color Space Conversion/1
  Green/1 -> Color Space Conversion/2
  Blue/1 -> Color Space Conversion/3
  Reshape/1 -> y1/1, y2/1
  Reshape1/1 -> u/1
  Reshape2/1 -> v/1
  Constant/1 -> y1/2
  Constant1/1 -> y2/2
  Constant2/1 -> u/2
  Constant3/1 -> v/2
  Transpose/1 -> Y1UY2VImage/1
  u/1 -> Matrix Concatenate/2
  y2/1 -> Matrix Concatenate/3
  Transpose1/1 -> Reshape/1
  Transpose2/1 -> Reshape1/1
  Transpose3/1 -> Reshape2/1
  " RGBImage "/1 -> Red/1
  "RGBImage "/1 -> Blue/1

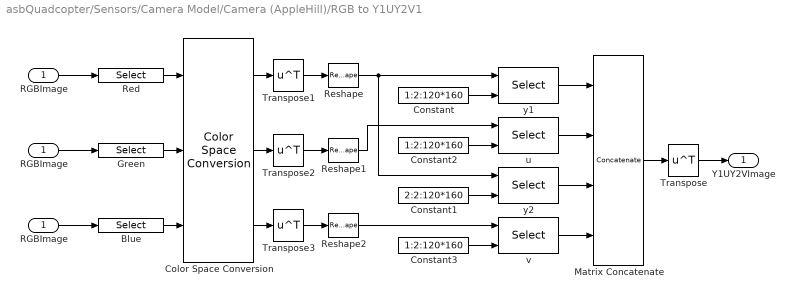
== system asbQuadcopter/Sensors/Camera Model/Camera (AppleHill)/RGB to Y1UY2V1 ==
  RGBImage : Inport  OutDataTypeStr=uint8  PortDimensions=[120 160 3]
  " RGBImage " : InportShadow  OutDataTypeStr=uint8  PortDimensions=[120 160 3]
  Blue : Selector  NumberOfDimensions=3  InputPortWidth=3  IndexOptions=Select all,Select all,Index vector (dialog)  Indices=1,1,3  OutputSizes=1,1,1
  Color Space Conversion : visionconversions/Color Space  Conversion  conversion=Obsolete  conversionActive=R'G'B' to Y'CbCr  wp_str=D65  rec=Rec. 601 (SDTV)  sys=1125/60/2:1  imagePorts=Separate color signals
  Constant : Constant  Value=1:2:120*160
  Constant1 : Constant  Value=2:2:120*160
  Constant2 : Constant  Value=1:2:120*160
  Constant3 : Constant  Value=1:2:120*160
  Green : Selector  NumberOfDimensions=3  InputPortWidth=3  IndexOptions=Select all,Select all,Index vector (dialog)  Indices=1,1,2  OutputSizes=1,1,1
  Matrix Concatenate : Concatenate  NumInputs=4  Mode=Multidimensional array  ConcatenateDimension=2
  "RGBImage " : InportShadow  OutDataTypeStr=uint8  PortDimensions=[120 160 3]
  Red : Selector  NumberOfDimensions=3  InputPortWidth=3  IndexOptions=Select all,Select all,Index vector (dialog)  Indices=1,1,1  OutputSizes=1,1,1
  Reshape : Reshape
  Reshape1 : Reshape
  Reshape2 : Reshape
  Transpose{,1..3} (4 alike) : Math  Operator=transpose  SignedPower=on
  u : Selector  InputPortWidth=120*160  IndexOptions=Index vector (port)  Indices=[1 3]  OutputSizes=1
  v : Selector  InputPortWidth=120*160  IndexOptions=Index vector (port)  Indices=[1 3]  OutputSizes=1
  y1 : Selector  InputPortWidth=120*160  IndexOptions=Index vector (port)  Indices=[1 3]  OutputSizes=1
  y2 : Selector  InputPortWidth=120*160  IndexOptions=Index vector (port)  Indices=[1 3]  OutputSizes=1
  Y1UY2VImage : Outport  OutDataTypeStr=uint8  PortDimensions=[4 9600]  VectorParamsAs1DForOutWhenUnconnected=off
  wires:
  Matrix Concatenate/1 -> Transpose/1
  v/1 -> Matrix Concatenate/4
  y1/1 -> Matrix Concatenate/1
  RGBImage/1 -> Green/1
  Color Space Conversion/2 -> Transpose2/1
  Color Space Conversion/1 -> Transpose1/1
  Color Space Conversion/3 -> Transpose3/1
  Red/1 -> Color Space Conversion/1
  Green/1 -> Color Space Conversion/2
  Blue/1 -> Color Space Conversion/3
  Reshape/1 -> y1/1, y2/1
  Reshape1/1 -> u/1
  Reshape2/1 -> v/1
  Constant/1 -> y1/2
  Constant1/1 -> y2/2
  Constant2/1 -> u/2
  Constant3/1 -> v/2
  Transpose/1 -> Y1UY2VImage/1
  u/1 -> Matrix Concatenate/2
  y2/1 -> Matrix Concatenate/3
  Transpose1/1 -> Reshape/1
  Transpose2/1 -> Reshape1/1
  Transpose3/1 -> Reshape2/1
  " RGBImage "/1 -> Red/1
  "RGBImage "/1 -> Blue/1

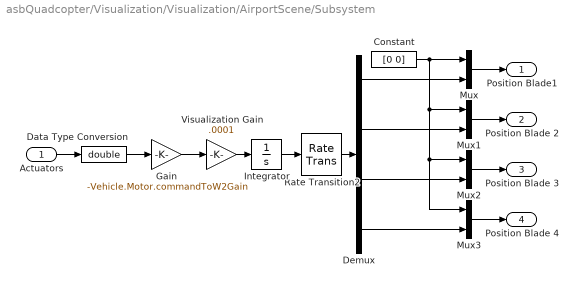
== system asbQuadcopter/Visualization/Visualization/AirportScene/Subsystem ==
  Actuators : Inport
  Constant : Constant  Value=[0 0]  VectorParams1D=off
  Data Type Conversion : DataTypeConversion  OutDataTypeStr=double  SaturateOnIntegerOverflow=off  RndMeth=Floor
  Demux : Demux
  Gain : Gain  Gain=-Vehicle.Motor.commandToW2Gain
  Integrator : Integrator  InitialCondition="[.1  .2 -.3 -.4]"  WrapState=on  WrappedStateUpperValue=2*pi  WrappedStateLowerValue=-2*pi
  Mux{,1..3} (4 alike) : Mux  Inputs=2
  Rate Transition2 : RateTransition
  Visualization Gain : Gain  Gain=.0001
  Position Blade1 : Outport  VectorParamsAs1DForOutWhenUnconnected=off
  Position Blade 2 : Outport  Port=2  VectorParamsAs1DForOutWhenUnconnected=off
  Position Blade 3 : Outport  Port=3  VectorParamsAs1DForOutWhenUnconnected=off
  Position Blade 4 : Outport  Port=4  VectorParamsAs1DForOutWhenUnconnected=off
  wires:
  Demux/4 -> Mux3/2
  Mux3/1 -> Position Blade 4/1
  Demux/2 -> Mux1/2
  Demux/3 -> Mux2/2
  Visualization Gain/1 -> Integrator/1
  Constant/1 -> Mux3/1, Mux2/1, Mux1/1, Mux/1
  Mux1/1 -> Position Blade 2/1
  Mux2/1 -> Position Blade 3/1
  Data Type Conversion/1 -> Gain/1
  Integrator/1 -> Rate Transition2/1
  Mux/1 -> Position Blade1/1
  Gain/1 -> Visualization Gain/1
  Demux/1 -> Mux/2
  Actuators/1 -> Data Type Conversion/1
  Rate Transition2/1 -> Demux/1
